simulink model "Inv_pendulum_cart_non_linear"  (R2022a)
settings: Solver=VariableStepAuto  StartTime=0.0  StopTime=40  RelTol=1e-3
values from neighbouring files (symbols this model uses):
  b = 0.02    [pendulum_cart.m]    (also in pendulum_cart_integral.m)
  g = 9.81    [pendulum_cart.m]    (also in pendulum_cart_integral.m)
  kv = 0.02    [pendulum_cart.m]    (also in pendulum_cart_integral.m)
  L = 1.0    (= 1)    [pendulum_cart.m]    (also in pendulum_cart_integral.m)
  M = 6.0    (= 6)    [pendulum_cart.m]    (also in pendulum_cart_integral.m)
  m = 1.5    [pendulum_cart.m]    (also in pendulum_cart_integral.m)
  Ts = 0.1    [pendulum_cart.m]    (also in pendulum_cart_integral.m)
undefined symbols (not defined in the file or in its folder): K
libraries: simulink x2
settings Model: Creator=Admin  LastModifiedBy=Admin

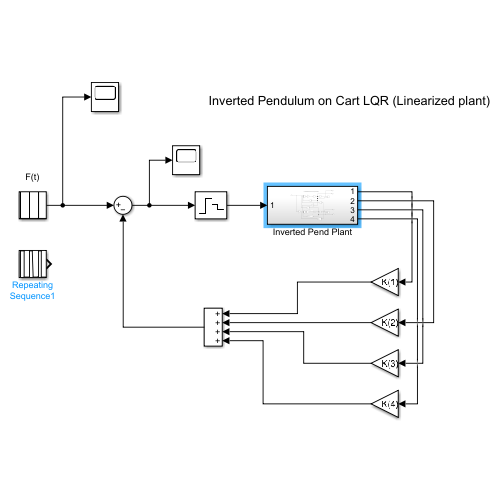
[thumbnail: Simulink's stored preview of the top-level diagram]
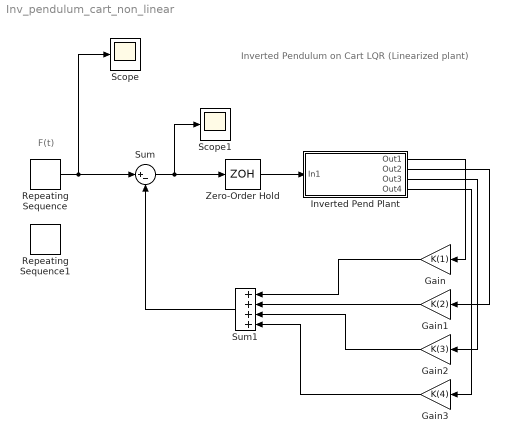
== system Inv_pendulum_cart_non_linear ==
  note: Inverted Pendulum on Cart LQR (Linearized plant)
  note: F(t)
  Gain : Gain  Gain=K(1)
  Gain1 : Gain  Gain=K(2)
  Gain2 : Gain  Gain=K(3)
  Gain3 : Gain  Gain=K(4)
  Inverted Pend Plant : Subsystem
  Repeating Sequence : simulink/Sources/Repeating Sequence  rep_seq_t="[0 2  2.1 2.25 2.30 50]"  rep_seq_y="[0 0  1    1   0    0]"
  Repeating Sequence1 : simulink/Sources/Repeating Sequence  rep_seq_t=[0 2 2.1 19 20 50]  rep_seq_y="[0 0 1    1   0    0]"
  Scope : Scope
  Scope1 : Scope
  Sum : Sum  Inputs=|+-
  Sum1 : Sum  Inputs=++++
  Zero-Order Hold : ZeroOrderHold  SampleTime=Ts
  wires:
  Repeating Sequence/1 -> Scope/1, Sum/1
  Sum1/1 -> Sum/2
  Gain/1 -> Sum1/1
  Gain1/1 -> Sum1/2
  Gain2/1 -> Sum1/3
  Gain3/1 -> Sum1/4
  Inverted Pend Plant/1(Out1) -> Gain/1
  Inverted Pend Plant/2(Out2) -> Gain1/1
  Inverted Pend Plant/3(Out3) -> Gain2/1
  Inverted Pend Plant/4(Out4) -> Gain3/1
  Zero-Order Hold/1 -> Inverted Pend Plant/1(In1)
  Sum/1 -> Scope1/1, Zero-Order Hold/1

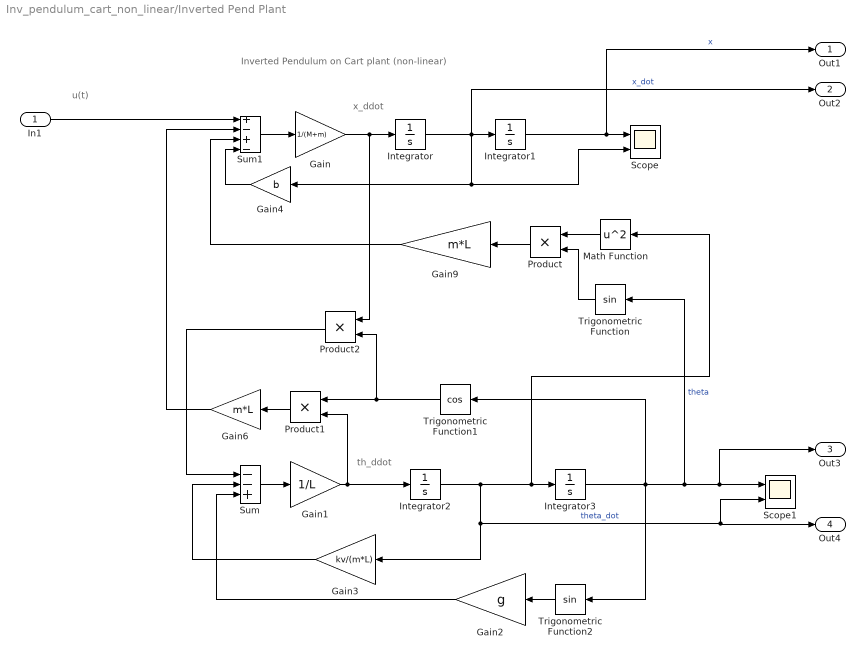
== system Inv_pendulum_cart_non_linear/Inverted Pend Plant ==
  note: x_ddot
  note: th_ddot
  note: Inverted Pendulum on Cart plant (non-linear)
  note: u(t)
  In1 : Inport
  Gain : Gain  Gain=1/(M+m)
  Gain1 : Gain  Gain=1/L
  Gain2 : Gain  Gain=g
  Gain3 : Gain  Gain=kv/(m*L)
  Gain4 : Gain  Gain=b
  Gain6 : Gain  Gain=m*L
  Gain9 : Gain  Gain=m*L
  Integrator : Integrator
  Integrator1 : Integrator
  Integrator2 : Integrator
  Integrator3 : Integrator  LimitOutput=on  UpperSaturationLimit=+1.1*pi  LowerSaturationLimit=-1.1*pi
  Math Function : Math  Operator=square
  Product : Product
  Product1 : Product
  Product2 : Product
  Scope : Scope  NumInputPorts=2
  Scope1 : Scope  NumInputPorts=2
  Sum : Sum  Inputs=--+
  Sum1 : Sum  Inputs=+-+-
  Trigonometric Function : Trigonometry
  Trigonometric Function1 : Trigonometry  Operator=cos
  Trigonometric Function2 : Trigonometry
  Out1 : Outport
  Out2 : Outport  Port=2
  Out3 : Outport  Port=3
  Out4 : Outport  Port=4
  wires:
  Integrator3/1 -> Trigonometric Function2/1, Trigonometric Function1/1, Out3/1, Scope1/1, Trigonometric Function/1  "theta"
  Sum/1 -> Gain1/1
  Gain/1 -> Product2/1, Integrator/1
  Gain2/1 -> Sum/3
  Gain1/1 -> Integrator2/1, Product1/2
  Integrator/1 -> Out2/1, Scope/2, Gain4/1, Integrator1/1  "x_dot"
  Gain6/1 -> Sum1/2
  Integrator1/1 -> Out1/1, Scope/1  "x"
  Integrator2/1 -> Gain3/1, Scope1/2, Out4/1, Math Function/1, Integrator3/1  "theta_dot"
  Gain4/1 -> Sum1/4
  Sum1/1 -> Gain/1
  In1/1 -> Sum1/1
  Trigonometric Function/1 -> Product/2
  Math Function/1 -> Product/1
  Product/1 -> Gain9/1
  Gain9/1 -> Sum1/3
  Trigonometric Function1/1 -> Product2/2, Product1/1
  Product1/1 -> Gain6/1
  Trigonometric Function2/1 -> Gain2/1
  Gain3/1 -> Sum/2
  Product2/1 -> Sum/1
